simulink model "Aeropendulum"  (Simulink 7.7)
settings: Solver=FixedStepDiscrete  StartTime=0.0  StopTime=60  RelTol=1e-3
undefined symbols (not defined in the file or in its folder): Serial_Port, Standard_Devices
libraries: rtwinlib x3, simulink x2, cstblocks x2
Description:
  | AeroPendulum Controller
  | -Phase lead
  | -Phase lag
  | -Proportional control
  | 
  | All controllers working!
settings Model: Creator=Josh Gill  LastModifiedBy=MEMS lab  SimulationMode=external  ExtModeEnableFloating=off  ExtModeTrigDuration=10000  ExtModeLogAll=off
settings DebuggingCC: StrictBusMsg=Warning
settings HardwareCC: ProdIntDivRoundTo=Zero  ProdEndianess=LittleEndian  ProdHWDeviceType=Generic->32-bit x86 compatible
settings RTWCC: SystemTargetFile=rtwin.tlc  TemplateMakefile=rtwin.tmf  Description=Real-Time Windows Target  ProcessScript=rtwin_make_rtw_hook  RTWCompilerOptimization=On
settings CodeAppCC: MaxIdLength=95
settings RTWinTargetCC: TargetLibSuffix=_rtwin.lib  TargetPreCompLibLocation=C:\Program Files\MATLAB\R2011a\toolbox\rtw\targets\rtwin\lib\win32  TargetFunctionLibrary=ANSI_C  FunctionExecutionProfile=off  CodeExecutionProfiling=off  ERTCodeCoverageTool=None  PortableWordSizes=off

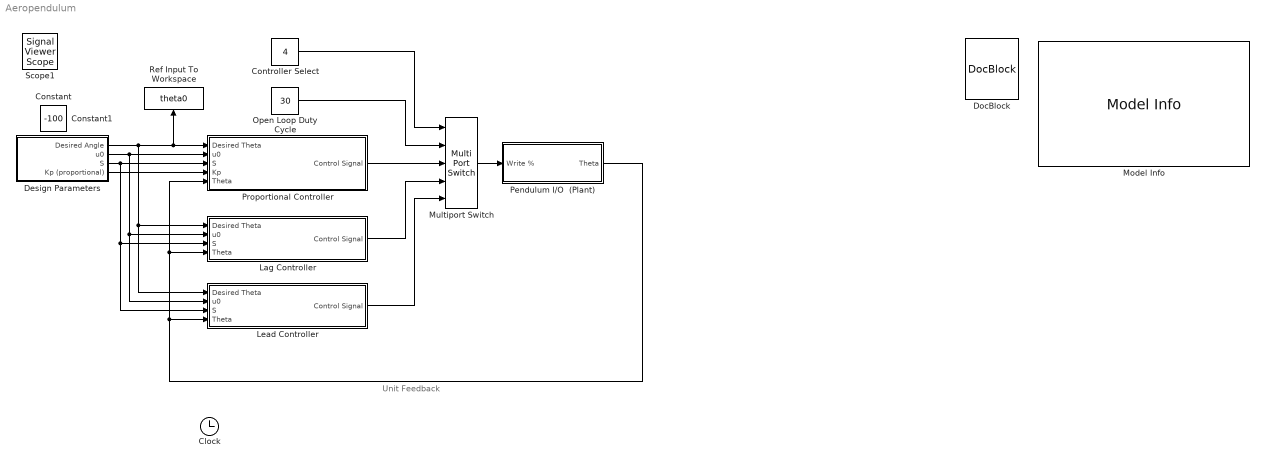
== system Aeropendulum ==
  note: Unit Feedback
  Controller Select : Constant  Value=4
  Design Parameters : Subsystem
  DocBlock : simulink/Model-Wide Utilities/DocBlock  SystemSampleTime=-1  DocumentType=Text
  Lag Controller : Subsystem
  Lead Controller : Subsystem
  Model Info : simulink/Model-Wide Utilities/Model Info  SystemSampleTime=-1  InitialBlockCM=None  BlockCM=None  Frame=on  DisplayStringWithTags=|  HorizontalTextAlignment=Center  LeftAlignmentValue=0.5  SourceBlockDiagram=Aeropendulum  TagMaxNumber=20
      | %<Description>
      | --------------------------------------
      | %<ModifiedBy>
      | %<ModifiedDate>
      | %<ModelVersion>
  Multiport Switch : MultiPortSwitch  Inputs=4  zeroidx=off
  Open Loop Duty Cycle : Constant  Value=30
  Pendulum I/O  (Plant) : Subsystem
  Proportional Controller : Subsystem
  "Ref Input To Workspace " : ToWorkspace  VariableName=theta0  SampleTime=-1  SaveFormat=Array
  Clock : Clock
      settings: IOType=siggen  Decimation=10
  Constant : Constant  IOType=siggen  Value=100
  Constant1 : Constant  IOType=siggen  Value=-100
  Scope1 : SignalViewerScope  IOType=viewer  ExtModeUploadOption=log  ZoomMode=yonly  LegendLocations="282.3333      221.3333           165            36"  RefreshTime=0.010417
      settings: TickLabels=on  ShowLegends=on  TimeRange=60  YMin=-50  YMax=140  SaveToWorkspace=on  MaxDataPoints=10000
  wires:
  Pendulum I/O  (Plant)/1(Theta) -> Proportional Controller/5(Theta), Lag Controller/4(Theta), Lead Controller/4(Theta)
  Design Parameters/1(Desired Angle) -> Lag Controller/1(Desired Theta), Lead Controller/1(Desired Theta), Proportional Controller/1(Desired Theta), "Ref Input To Workspace "/1
  Design Parameters/3(S) -> Proportional Controller/3(S), Lag Controller/3(S), Lead Controller/3(S)
  Multiport Switch/1 -> Pendulum I/O  (Plant)/1(Write %)
  Open Loop Duty Cycle/1 -> Multiport Switch/2
  Design Parameters/2(u0) -> Proportional Controller/2(u0), Lag Controller/2(u0), Lead Controller/2(u0)
  Design Parameters/4(Kp (proportional)) -> Proportional Controller/4(Kp)
  Proportional Controller/1(Control Signal) -> Multiport Switch/3
  Lag Controller/1(Control Signal) -> Multiport Switch/4
  Lead Controller/1(Control Signal) -> Multiport Switch/5
  Controller Select/1 -> Multiport Switch/1

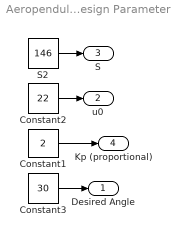
== system Aeropendulum/Design Parameters ==
  Constant1 : Constant  Value=2
  Constant2 : Constant  Value=22
  Constant3 : Constant  Value=30
  S2 : Constant  Value=146
  Desired Angle : Outport
  u0 : Outport  Port=2
  S : Outport  Port=3
  Kp (proportional) : Outport  Port=4
  wires:
  Constant2/1 -> u0/1
  Constant1/1 -> Kp (proportional)/1
  Constant3/1 -> Desired Angle/1
  S2/1 -> S/1

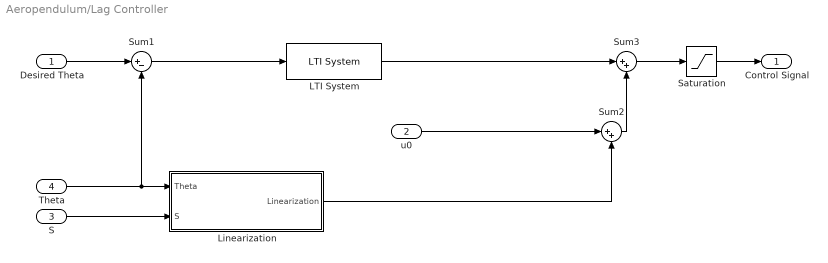
== system Aeropendulum/Lag Controller ==
  Desired Theta : Inport
  u0 : Inport  Port=2
  S : Inport  Port=3
  Theta : Inport  Port=4
  LTI System : cstblocks/LTI System  SystemSampleTime=-1  sys=clagd  IC=[]
  Linearization : Subsystem
  Saturation : Saturate  UpperLimit=127  LowerLimit=-127
  Sum1 : Sum  Inputs=|+-
  Sum2 : Sum  Inputs=|++
  Sum3 : Sum  Inputs=|++
  Control Signal : Outport
  wires:
  Theta/1 -> Linearization/1(Theta), Sum1/2
  Desired Theta/1 -> Sum1/1
  Sum3/1 -> Saturation/1
  Sum1/1 -> LTI System/1
  u0/1 -> Sum2/1
  Saturation/1 -> Control Signal/1
  LTI System/1 -> Sum3/1
  Sum2/1 -> Sum3/2
  Linearization/1(Linearization) -> Sum2/2
  S/1 -> Linearization/2(S)

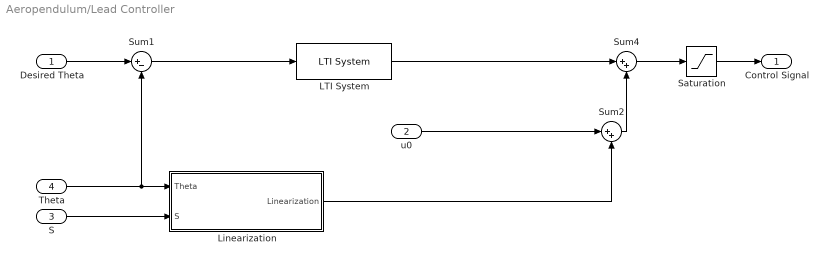
== system Aeropendulum/Lead Controller ==
  Desired Theta : Inport
  u0 : Inport  Port=2
  S : Inport  Port=3
  Theta : Inport  Port=4
  LTI System : cstblocks/LTI System  SystemSampleTime=-1  sys=clead  IC=[]
  Linearization : Subsystem
  Saturation : Saturate  UpperLimit=127  LowerLimit=-127
  Sum1 : Sum  Inputs=|+-
  Sum2 : Sum  Inputs=|++
  Sum4 : Sum  Inputs=|++
  Control Signal : Outport
  wires:
  Theta/1 -> Linearization/1(Theta), Sum1/2
  Desired Theta/1 -> Sum1/1
  Sum4/1 -> Saturation/1
  u0/1 -> Sum2/1
  Saturation/1 -> Control Signal/1
  Sum2/1 -> Sum4/2
  Linearization/1(Linearization) -> Sum2/2
  S/1 -> Linearization/2(S)
  Sum1/1 -> LTI System/1
  LTI System/1 -> Sum4/1

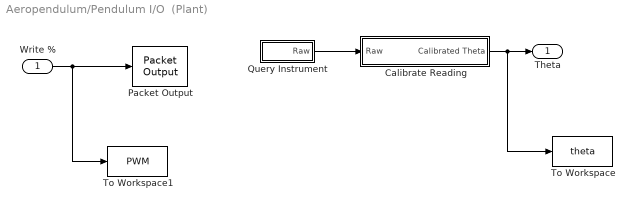
== system Aeropendulum/Pendulum I/O  (Plant) ==
  Write % : Inport
  Calibrate Reading : Subsystem
  Packet Output : rtwinlib/Packet Output  SampleTime=-1  DrvName=Standard_Devices/Serial_Port  DrvAddress=4  DrvOptions=[9600 8 0 0 0 0 0 0]  PacketSize=1  DataTypes='int8'  ShowReady=off  ShowError=off  PacketID=1  ByteOrder=1  InitialValue=[]  FinalValue=[]
      settings: AttributesFormatString=Standard Devices\nSerial Port [4h]
  Query Instrument : Subsystem
  To Workspace : ToWorkspace  VariableName=theta  SampleTime=-1  SaveFormat=Array
  To Workspace1 : ToWorkspace  VariableName=PWM  SampleTime=-1  SaveFormat=Array
  Theta : Outport
  wires:
  Write %/1 -> Packet Output/1, To Workspace1/1
  Query Instrument/1(Raw) -> Calibrate Reading/1(Raw)
  Calibrate Reading/1(Calibrated Theta) -> Theta/1, To Workspace/1

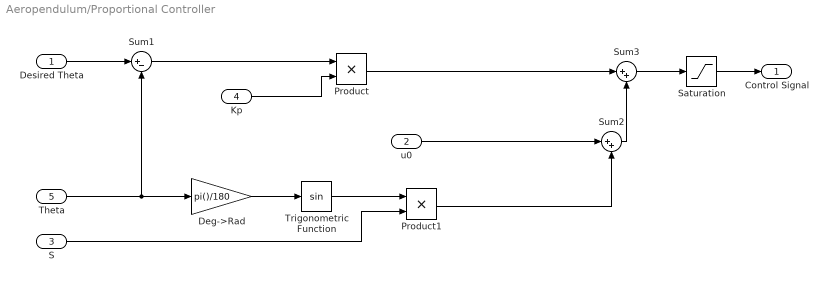
== system Aeropendulum/Proportional Controller ==
  Desired Theta : Inport
  u0 : Inport  Port=2
  S : Inport  Port=3
  Kp : Inport  Port=4
  Theta : Inport  Port=5
  Deg->Rad : Gain  Gain=pi()/180
  Product : Product  RndMeth=Zero
  Product1 : Product  RndMeth=Zero
  Saturation : Saturate  UpperLimit=127  LowerLimit=-127
  Sum1 : Sum  Inputs=|+-
  Sum2 : Sum  Inputs=|++
  Sum3 : Sum  Inputs=|++
  Trigonometric Function : Trigonometry
  Control Signal : Outport
  wires:
  Theta/1 -> Sum1/2, Deg->Rad/1
  Desired Theta/1 -> Sum1/1
  Sum3/1 -> Saturation/1
  Sum1/1 -> Product/1
  u0/1 -> Sum2/1
  Saturation/1 -> Control Signal/1
  Product/1 -> Sum3/1
  Sum2/1 -> Sum3/2
  Kp/1 -> Product/2
  Trigonometric Function/1 -> Product1/1
  Deg->Rad/1 -> Trigonometric Function/1
  Product1/1 -> Sum2/2
  S/1 -> Product1/2

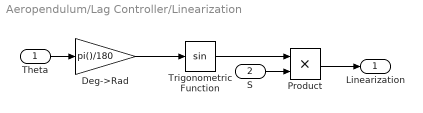
== system Aeropendulum/Lag Controller/Linearization ==
  Theta : Inport
  S : Inport  Port=2
  Deg->Rad : Gain  Gain=pi()/180
  Product : Product  RndMeth=Zero
  Trigonometric Function : Trigonometry
  Linearization : Outport
  wires:
  Trigonometric Function/1 -> Product/1
  Deg->Rad/1 -> Trigonometric Function/1
  Theta/1 -> Deg->Rad/1
  Product/1 -> Linearization/1
  S/1 -> Product/2

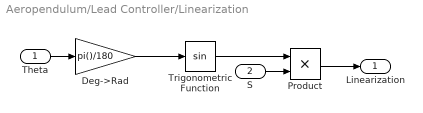
== system Aeropendulum/Lead Controller/Linearization ==
  Theta : Inport
  S : Inport  Port=2
  Deg->Rad : Gain  Gain=pi()/180
  Product : Product  RndMeth=Zero
  Trigonometric Function : Trigonometry
  Linearization : Outport
  wires:
  Trigonometric Function/1 -> Product/1
  Deg->Rad/1 -> Trigonometric Function/1
  Theta/1 -> Deg->Rad/1
  Product/1 -> Linearization/1
  S/1 -> Product/2

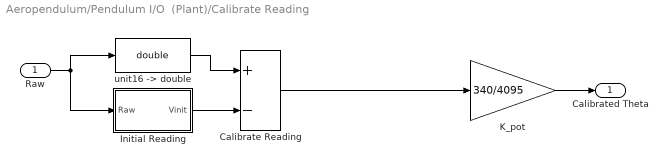
== system Aeropendulum/Pendulum I/O  (Plant)/Calibrate Reading ==
  Raw : Inport
  Calibrate Reading : Sum  Inputs=+-
  Initial Reading : Subsystem
  K_pot : Gain  Gain=340/4095  OutDataTypeStr=Inherit: Inherit via back propagation  SaturateOnIntegerOverflow=on
  "unit16 -> double" : DataTypeConversion  OutDataTypeStr=double
  Calibrated Theta : Outport
  wires:
  Initial Reading/1(Vinit) -> Calibrate Reading/2
  Raw/1 -> Initial Reading/1(Raw), "unit16 -> double"/1
  Calibrate Reading/1 -> K_pot/1
  K_pot/1 -> Calibrated Theta/1
  "unit16 -> double"/1 -> Calibrate Reading/1

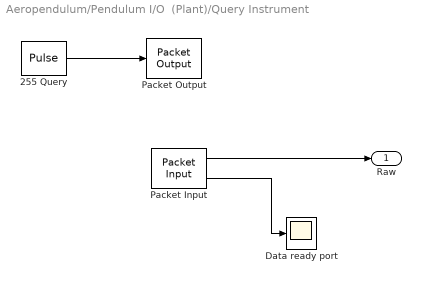
== system Aeropendulum/Pendulum I/O  (Plant)/Query Instrument ==
  255 Query : DiscretePulseGenerator  PulseType=Time based  Amplitude=128  Period=.02  PulseWidth=50
  Data ready port : Scope
      settings: YMin=0  YMax=1  SaveName=ScopeData3
  Packet Input : rtwinlib/Packet Input  SampleTime=.01  DrvName=Standard_Devices/Serial_Port  DrvAddress=4  DrvOptions=[9600 8 0 0 0 0 0 0]  PacketSize=2  DataTypes='uint16'  ShowReady=on  ShowError=off  PacketID=1  ByteOrder=1  ShowTimestamp=off
      settings: AttributesFormatString=Standard Devices\nSerial Port [4h]
  Packet Output : rtwinlib/Packet Output  SampleTime=-1  DrvName=Standard_Devices/Serial_Port  DrvAddress=4  DrvOptions=[9600 8 0 0 0 0 0 0]  PacketSize=1  DataTypes='int8'  ShowReady=off  ShowError=off  PacketID=1  ByteOrder=1  InitialValue=[]  FinalValue=[]
      settings: AttributesFormatString=Standard Devices\nSerial Port [4h]
  Raw : Outport
  wires:
  255 Query/1 -> Packet Output/1
  Packet Input/2 -> Data ready port/1
  Packet Input/1 -> Raw/1

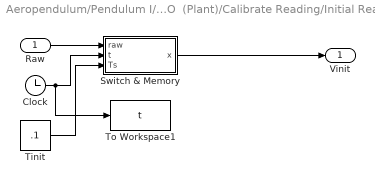
== system Aeropendulum/Pendulum I/O  (Plant)/Calibrate Reading/Initial Reading ==
  Raw : Inport
  Clock : Clock
      settings: Decimation=10
  Switch & Memory : Stateflow chart  TreatAsAtomicUnit=on
  Tinit : Constant  Value=.1
  To Workspace1 : ToWorkspace  VariableName=t  SampleTime=-1  SaveFormat=Array
  Vinit : Outport
  wires:
  Clock/1 -> Switch & Memory/2(t), To Workspace1/1
  Tinit/1 -> Switch & Memory/3(Ts)
  Raw/1 -> Switch & Memory/1(raw)
  Switch & Memory/1(x) -> Vinit/1

== matlab function Pendulum I/O (Plant)/Calibrate Reading/Initial Reading/Switch & Memory ==
  data: x output double; raw input double; t input double; Ts input double

function x = fcn(raw,t, Ts)

    %memorize initial position
    persistent xy;
      
    %if time is less than time to acquire signal, save.
    if(isempty(xy) || t < Ts)

            xy = raw;

    end
    
    %return value
    x = xy;
    
    
end
